simulink model "Sylvester_sym"  (R2020a)
settings: Solver=FixedStepAuto  StartTime=0.0  StopTime=t  FixedStep=0.01  RelTol=1e-3
values from neighbouring files (symbols this model uses):
  A = [-0.0226 -36.6 -18.9 -32.1 ;            0 -1.9  0.983     0;       0.0123 -11.7 -2.63     0;            0     0     1     0]    [Sylvester.m]
  B = [0      0;      -0.414 0;      -77.8 22.4;      0     0]    [Sylvester.m]
  C = [0  57.3  0  0;      0    0   0  57.3]    [Sylvester.m]
  D = zeros(2,2)    [Sylvester.m]
  inpt = 1    [Sylvester.m]
  L = ones(4,2)    [Sylvester.m]
  M = eye(4)*diag([-6 -5 -7 -8])    [Sylvester.m]
  N = double(nT*B-L*D)    [Sylvester.m]
  nT = double([cT(1) cT(2) cT(3) cT(4);       cT(5) cT(6) cT(7) cT(8);       cT(9) cT(10) cT(11) cT(12);       cT(13) cT(14) cT(15) cT(16)])    [Sylvester.m]
  x0 = [1 1 1 1]'    [Sylvester.m]
  z0 = nT*[-1 -1 -1 -1]'    [Sylvester.m]
undefined symbols (not defined in the file or in its folder): sigbuilder_block
settings Model: Creator=grzyb  LastModifiedBy=grzyb

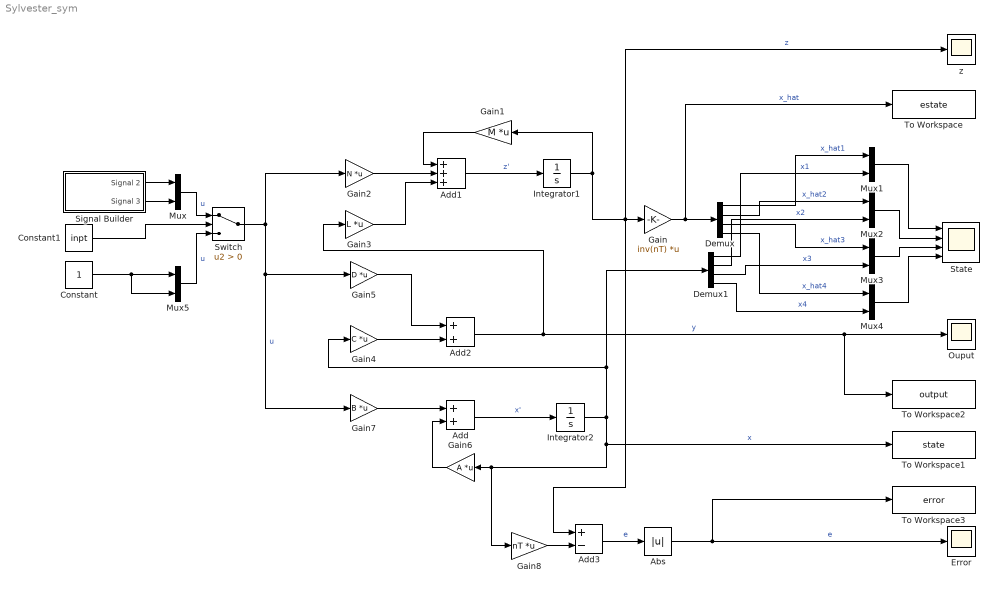
== system Sylvester_sym ==
  Abs : Abs
  Add : Sum
  Add1 : Sum  Inputs=+++
  Add2 : Sum
  Add3 : Sum  Inputs=+-
  Constant : Constant
  Constant1 : Constant  Value=inpt
  Demux : Demux
  Demux1 : Demux
  Error : Scope
  Gain : Gain  Gain=inv(nT)  Multiplication=Matrix(K*u)
  Gain1 : Gain  Gain=M  Multiplication=Matrix(K*u)
  Gain2 : Gain  Gain=N  Multiplication=Matrix(K*u)
  Gain3 : Gain  Gain=L  Multiplication=Matrix(K*u)
  Gain4 : Gain  Gain=C  Multiplication=Matrix(K*u)
  Gain5 : Gain  Gain=D  Multiplication=Matrix(K*u)
  Gain6 : Gain  Gain=A  Multiplication=Matrix(K*u)
  Gain7 : Gain  Gain=B  Multiplication=Matrix(K*u)
  Gain8 : Gain  Gain=nT  Multiplication=Matrix(K*u)
  Integrator1 : Integrator  InitialCondition=z0
  Integrator2 : Integrator  InitialCondition=x0
  Mux{,1..5} (6 alike) : Mux  Inputs=2
  Ouput : Scope
  Signal Builder : Subsystem  Tag=STV Subsys  LoadFcn=sigbuilder_block('load');  StartFcn=sigbuilder_block('start');  StopFcn=sigbuilder_block('stop');  ClipboardFcn=sigbuilder_block('clipboard');  mask(Sigbuilder block){tuvar=[0:10]}
      mask help: Simulink:masks:SigbuilderBlock_MD
      mask init:
      | if ~strcmp(get_param(bdroot(gcbh),'SimulationStatus'),'stopped') tuvar = sigbuilder_block('maskInit'); end
      settings: CopyFcn=sigbuilder_block('copy');  DeleteFcn=sigbuilder_block('delete');  ModelCloseFcn=sigbuilder_block('modelClose');  PreSaveFcn=sigbuilder_block('preSave');  PauseFcn=sigbuilder_block('pause');  ContinueFcn=sigbuilder_block('continue');  NameChangeFcn=sigbuilder_block('namechange');  OpenFcn=sigbuilder_block('open',[437.6 199.2 550.4 400 ]);  CloseFcn=sigbuilder_block('close');
      mask Display: plot(0, 0, 100, 100,[2, 2, 32, 32, 2], [68, 8, 8, 68, 68],[32, 2], [38, 38], [32, 19, 2],[53, 60, 44], [32, 17, 17, 2],[16, 16, 31, 31]);txt = getActiveGroup(gcbh);text(2, 100, txt,'verticalAlignment', 'top');
  State : Scope  NumInputPorts=4
  Switch : Switch  Criteria=u2 > Threshold
  To Workspace : ToWorkspace  VariableName=estate  SaveFormat=Structure  SampleTime=-1
  To Workspace1 : ToWorkspace  VariableName=state  SaveFormat=Structure  SampleTime=-1
  To Workspace2 : ToWorkspace  VariableName=output  SaveFormat=Structure  SampleTime=-1
  To Workspace3 : ToWorkspace  VariableName=error  SaveFormat=Structure  SampleTime=-1
  z : Scope
  wires:
  Add1/1 -> Integrator1/1  "z'"
  Gain1/1 -> Add1/1
  Integrator1/1 -> z/1, Gain/1, Add3/1, Gain1/1  "z"
  Gain2/1 -> Add1/2
  Switch/1 -> Gain2/1, Gain7/1, Gain5/1  "u"
  Gain3/1 -> Add1/3
  Add2/1 -> To Workspace2/1, Ouput/1, Gain3/1  "y"
  Gain4/1 -> Add2/2
  Gain5/1 -> Add2/1
  Add/1 -> Integrator2/1  "x'"
  Integrator2/1 -> To Workspace1/1, Gain8/1, Gain6/1, Demux1/1, Gain4/1  "x"
  Gain6/1 -> Add/2
  Gain7/1 -> Add/1
  Add3/1 -> Abs/1  "e"
  Gain8/1 -> Add3/2
  Gain/1 -> Demux/1, To Workspace/1  "x_hat"
  Mux1/1 -> State/1
  Mux2/1 -> State/2
  Mux3/1 -> State/3
  Mux4/1 -> State/4
  Demux/1 -> Mux1/1  "x_hat1"
  Demux/2 -> Mux2/1  "x_hat2"
  Demux/3 -> Mux3/1  "x_hat3"
  Demux/4 -> Mux4/1  "x_hat4"
  Demux1/1 -> Mux1/2  "x1"
  Demux1/2 -> Mux2/2  "x2"
  Demux1/3 -> Mux3/2  "x3"
  Demux1/4 -> Mux4/2  "x4"
  Abs/1 -> To Workspace3/1, Error/1  "e"
  Signal Builder/1(Signal 2) -> Mux/1
  Signal Builder/2(Signal 3) -> Mux/2
  Mux/1 -> Switch/1  "u"
  Constant/1 -> Mux5/2, Mux5/1
  Mux5/1 -> Switch/3  "u"
  Constant1/1 -> Switch/2

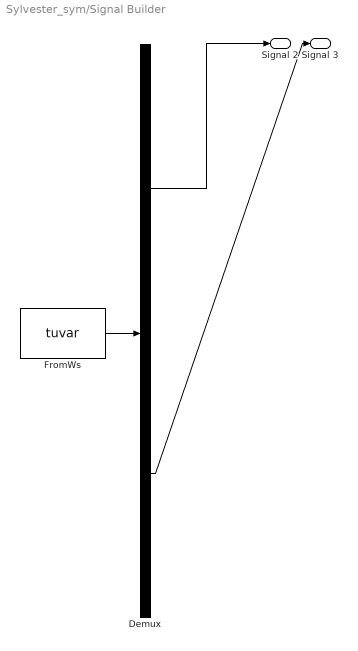
== system Sylvester_sym/Signal Builder ==
  Demux : Demux  Tag=STV Demux  Outputs=2
      settings: DisplayOption=none
  FromWs : FromWorkspace  Tag=STV FromWs  VariableName=tuvar
      SigBuilderData=|
      | common.afterFinalStr = 'Extrapolate'
      | common.sampleTime = 0
      | dataSet.timeRange = [0 10]
      | dataSet.name = 'Group 1'
      | sbobj.Groups.Name = 'Group 1'
      | sbobj.Groups.Signals(1).Name = 'Signal 2'
      | sbobj.Groups.Signals(1).XData = [0 2 2 10]
      | sbobj.Groups.Signals(1).YData = [0 0 1 1]
      | sbobj.Groups.Signals(2).Name = 'Signal 3'
      | sbobj.Groups.Signals(2).XData = [0 7 7 10]
      | sbobj.Groups.Signals(2).YData = [0 0 1 1]
  Signal 2 : Outport  Tag=STV Outport
  Signal 3 : Outport  Tag=STV Outport  Port=2
  wires:
  FromWs/1 -> Demux/1
  Demux/1 -> Signal 2/1
  Demux/2 -> Signal 3/1
